simulink model "ASM_Traffic_V2X_Complete_Model_2"  (R2019a)
settings: Solver=ode1  StartTime=SIM.tstart.v  StopTime=Inf  FixedStep=SIM.StepSize.v  RelTol=1e-3
PostLoadFcn:
  | if any(exist('dsrtsu_mdlpostloadfcn', 'file') ~= 0), dsrtsu_mdlpostloadfcn('Execute', bdroot); end
  | try, asm_mdl_postloadfcn(bdroot, 'UpdateModel', 2200); catch, disp(lasterr); end,
undefined symbols (not defined in the file): _SensorPnts_1, _SensorPnts_13, _SensorPnts_17, _SensorPnts_21, _SensorPnts_25, _SensorPnts_29, _SensorPnts_33, _SensorPnts_37, _SensorPnts_41, _SensorPnts_45, _SensorPnts_49, _SensorPnts_5, _SensorPnts_53, _SensorPnts_57, _SensorPnts_9, _to_, CPT, G5A, ITS, MDL, rad, s_to_rpm, SIM
libraries: simulink x169, ASM_VehicleDynamics_lib x126, ASM_Traffic_lib x83, ASM_Utils_lib x49, mdbs x45, ASM_Environment_lib x17, dspindex x12, dsaV2xLibraryAux x10, dsmpblib x6, dsaV2xAsn1Library x4, dsaV2xLibrary x4, ASM_BrakeHydraulics_lib x4
(part 33 of 36)

== system ASM_Traffic_V2X_Complete_Model_2/MDLUserInterface/Environment/MDL_DISP/Traffic/Object_Sensor_2D/IdxSelect_2DSensor/Scopezone_Element_Data_Selection3/Object_Type[]1 ==
  In1 : Inport
  Out1 : Outport
  wires:
  In1/1 -> Out1/1

== system ASM_Traffic_V2X_Complete_Model_2/MDLUserInterface/Environment/MDL_DISP/Traffic/Object_Sensor_2D/IdxSelect_2DSensor/Scopezone_Element_Data_Selection3/a_Rel[m|s2]1 ==
  In1 : Inport
  Out1 : Outport
  wires:
  In1/1 -> Out1/1

== system ASM_Traffic_V2X_Complete_Model_2/MDLUserInterface/Environment/MDL_DISP/Traffic/Object_Sensor_2D/IdxSelect_2DSensor/Scopezone_Element_Data_Selection3/v_Rel[m|s]1 ==
  In1 : Inport
  Out1 : Outport
  wires:
  In1/1 -> Out1/1

== system ASM_Traffic_V2X_Complete_Model_2/MDLUserInterface/Environment/MDL_DISP/Traffic/Object_Sensor_2D/IdxSelect_2DSensor/Scopezone_Element_Data_Selection4/Angle_Hor_Rel[deg]1 ==
  In1 : Inport
  Out1 : Outport
  wires:
  In1/1 -> Out1/1

== system ASM_Traffic_V2X_Complete_Model_2/MDLUserInterface/Environment/MDL_DISP/Traffic/Object_Sensor_2D/IdxSelect_2DSensor/Scopezone_Element_Data_Selection4/Distance[m]1 ==
  In1 : Inport
  Out1 : Outport
  wires:
  In1/1 -> Out1/1

== system ASM_Traffic_V2X_Complete_Model_2/MDLUserInterface/Environment/MDL_DISP/Traffic/Object_Sensor_2D/IdxSelect_2DSensor/Scopezone_Element_Data_Selection4/Flag_Object_In_Scope[0Out|1In]1 ==
  In1 : Inport
  Out1 : Outport
  wires:
  In1/1 -> Out1/1

== system ASM_Traffic_V2X_Complete_Model_2/MDLUserInterface/Environment/MDL_DISP/Traffic/Object_Sensor_2D/IdxSelect_2DSensor/Scopezone_Element_Data_Selection4/Flag_Sensor_Apex_In_Object[0Out|1In]1 ==
  In1 : Inport
  Out1 : Outport
  wires:
  In1/1 -> Out1/1

== system ASM_Traffic_V2X_Complete_Model_2/MDLUserInterface/Environment/MDL_DISP/Traffic/Object_Sensor_2D/IdxSelect_2DSensor/Scopezone_Element_Data_Selection4/Height_Max[m]1 ==
  In1 : Inport
  Out1 : Outport
  wires:
  In1/1 -> Out1/1

== system ASM_Traffic_V2X_Complete_Model_2/MDLUserInterface/Environment/MDL_DISP/Traffic/Object_Sensor_2D/IdxSelect_2DSensor/Scopezone_Element_Data_Selection4/Height_Min[m]1 ==
  In1 : Inport
  Out1 : Outport
  wires:
  In1/1 -> Out1/1

== system ASM_Traffic_V2X_Complete_Model_2/MDLUserInterface/Environment/MDL_DISP/Traffic/Object_Sensor_2D/IdxSelect_2DSensor/Scopezone_Element_Data_Selection4/Object_ID[]1 ==
  In1 : Inport
  Out1 : Outport
  wires:
  In1/1 -> Out1/1

== system ASM_Traffic_V2X_Complete_Model_2/MDLUserInterface/Environment/MDL_DISP/Traffic/Object_Sensor_2D/IdxSelect_2DSensor/Scopezone_Element_Data_Selection4/Object_Type[]1 ==
  In1 : Inport
  Out1 : Outport
  wires:
  In1/1 -> Out1/1

== system ASM_Traffic_V2X_Complete_Model_2/MDLUserInterface/Environment/MDL_DISP/Traffic/Object_Sensor_2D/IdxSelect_2DSensor/Scopezone_Element_Data_Selection4/a_Rel[m|s2]1 ==
  In1 : Inport
  Out1 : Outport
  wires:
  In1/1 -> Out1/1

== system ASM_Traffic_V2X_Complete_Model_2/MDLUserInterface/Environment/MDL_DISP/Traffic/Object_Sensor_2D/IdxSelect_2DSensor/Scopezone_Element_Data_Selection4/v_Rel[m|s]1 ==
  In1 : Inport
  Out1 : Outport
  wires:
  In1/1 -> Out1/1

== system ASM_Traffic_V2X_Complete_Model_2/MDLUserInterface/Environment/MDL_DISP/Traffic/Object_Sensor_2D/IdxSelect_2DSensor/Scopezone_Element_Data_Selection5/Angle_Hor_Rel[deg]1 ==
  In1 : Inport
  Out1 : Outport
  wires:
  In1/1 -> Out1/1

== system ASM_Traffic_V2X_Complete_Model_2/MDLUserInterface/Environment/MDL_DISP/Traffic/Object_Sensor_2D/IdxSelect_2DSensor/Scopezone_Element_Data_Selection5/Distance[m]1 ==
  In1 : Inport
  Out1 : Outport
  wires:
  In1/1 -> Out1/1

== system ASM_Traffic_V2X_Complete_Model_2/MDLUserInterface/Environment/MDL_DISP/Traffic/Object_Sensor_2D/IdxSelect_2DSensor/Scopezone_Element_Data_Selection5/Flag_Object_In_Scope[0Out|1In]1 ==
  In1 : Inport
  Out1 : Outport
  wires:
  In1/1 -> Out1/1

== system ASM_Traffic_V2X_Complete_Model_2/MDLUserInterface/Environment/MDL_DISP/Traffic/Object_Sensor_2D/IdxSelect_2DSensor/Scopezone_Element_Data_Selection5/Flag_Sensor_Apex_In_Object[0Out|1In]1 ==
  In1 : Inport
  Out1 : Outport
  wires:
  In1/1 -> Out1/1

== system ASM_Traffic_V2X_Complete_Model_2/MDLUserInterface/Environment/MDL_DISP/Traffic/Object_Sensor_2D/IdxSelect_2DSensor/Scopezone_Element_Data_Selection5/Height_Max[m]1 ==
  In1 : Inport
  Out1 : Outport
  wires:
  In1/1 -> Out1/1

== system ASM_Traffic_V2X_Complete_Model_2/MDLUserInterface/Environment/MDL_DISP/Traffic/Object_Sensor_2D/IdxSelect_2DSensor/Scopezone_Element_Data_Selection5/Height_Min[m]1 ==
  In1 : Inport
  Out1 : Outport
  wires:
  In1/1 -> Out1/1

== system ASM_Traffic_V2X_Complete_Model_2/MDLUserInterface/Environment/MDL_DISP/Traffic/Object_Sensor_2D/IdxSelect_2DSensor/Scopezone_Element_Data_Selection5/Object_ID[]1 ==
  In1 : Inport
  Out1 : Outport
  wires:
  In1/1 -> Out1/1

== system ASM_Traffic_V2X_Complete_Model_2/MDLUserInterface/Environment/MDL_DISP/Traffic/Object_Sensor_2D/IdxSelect_2DSensor/Scopezone_Element_Data_Selection5/Object_Type[]1 ==
  In1 : Inport
  Out1 : Outport
  wires:
  In1/1 -> Out1/1

== system ASM_Traffic_V2X_Complete_Model_2/MDLUserInterface/Environment/MDL_DISP/Traffic/Object_Sensor_2D/IdxSelect_2DSensor/Scopezone_Element_Data_Selection5/a_Rel[m|s2]1 ==
  In1 : Inport
  Out1 : Outport
  wires:
  In1/1 -> Out1/1

== system ASM_Traffic_V2X_Complete_Model_2/MDLUserInterface/Environment/MDL_DISP/Traffic/Object_Sensor_2D/IdxSelect_2DSensor/Scopezone_Element_Data_Selection5/v_Rel[m|s]1 ==
  In1 : Inport
  Out1 : Outport
  wires:
  In1/1 -> Out1/1

== system ASM_Traffic_V2X_Complete_Model_2/MDLUserInterface/Environment/MDL_DISP/Traffic/Traffic_Sign_Sensor/GetTrfSgnDataByIndex_1/SwitchObjectPosition/Idx_comp ==
  Idx : Inport
  Add : Sum
  Add1 : Sum  Inputs=+-
  Add2 : Sum
  Add3 : Sum
  Constant : Constant
  Constant1 : Constant
  Constant2 : Constant  Value=2
  Constant3 : Constant  Value=3
  Gain : Gain  Gain=3
  Idx_comp_x : Outport
  Idx_comp_y : Outport  Port=2
  Idx_comp_z : Outport  Port=3
  wires:
  Constant/1 -> Add/2
  Idx/1 -> Add1/1
  Constant1/1 -> Add1/2
  Add1/1 -> Gain/1
  Gain/1 -> Add3/1, Add2/1, Add/1
  Add/1 -> Idx_comp_x/1
  Constant2/1 -> Add2/2
  Constant3/1 -> Add3/2
  Add2/1 -> Idx_comp_y/1
  Add3/1 -> Idx_comp_z/1

== system ASM_Traffic_V2X_Complete_Model_2/MDLUserInterface/Environment/MDL_DISP/Traffic/Traffic_Sign_Sensor/GetTrfSgnDataByIndex_1/SwitchObjectPosition/Idx_comp1 ==
  Idx : Inport
  Add : Sum
  Add1 : Sum  Inputs=+-
  Add2 : Sum
  Add3 : Sum
  Constant : Constant
  Constant1 : Constant
  Constant2 : Constant  Value=2
  Constant3 : Constant  Value=3
  Gain : Gain  Gain=3
  Idx_comp_x : Outport
  Idx_comp_y : Outport  Port=2
  Idx_comp_z : Outport  Port=3
  wires:
  Add3/1 -> Idx_comp_z/1
  Add2/1 -> Idx_comp_y/1
  Constant3/1 -> Add3/2
  Constant2/1 -> Add2/2
  Add/1 -> Idx_comp_x/1
  Gain/1 -> Add/1, Add2/1, Add3/1
  Add1/1 -> Gain/1
  Constant1/1 -> Add1/2
  Idx/1 -> Add1/1
  Constant/1 -> Add/2

== system ASM_Traffic_V2X_Complete_Model_2/MDLUserInterface/Environment/MDL_DISP/Traffic/Traffic_Sign_Sensor/GetTrfSgnDataByIndex_1/SwitchObjectPosition/Idx_comp2 ==
  Idx : Inport
  Add : Sum
  Add1 : Sum  Inputs=+-
  Add2 : Sum
  Add3 : Sum
  Constant : Constant
  Constant1 : Constant
  Constant2 : Constant  Value=2
  Constant3 : Constant  Value=3
  Gain : Gain  Gain=3
  Idx_comp_x : Outport
  Idx_comp_y : Outport  Port=2
  Idx_comp_z : Outport  Port=3
  wires:
  Constant/1 -> Add/2
  Idx/1 -> Add1/1
  Constant1/1 -> Add1/2
  Add1/1 -> Gain/1
  Gain/1 -> Add3/1, Add2/1, Add/1
  Add/1 -> Idx_comp_x/1
  Constant2/1 -> Add2/2
  Constant3/1 -> Add3/2
  Add2/1 -> Idx_comp_y/1
  Add3/1 -> Idx_comp_z/1

== system ASM_Traffic_V2X_Complete_Model_2/MDLUserInterface/Environment/MDL_DISP/Traffic/Traffic_Sign_Sensor/GetTrfSgnDataByIndex_1/SwitchSignProperties/Idx_comp ==
  Idx : Inport
  Add{,2..5} (5 alike) : Sum
  Add1 : Sum  Inputs=+-
  Constant : Constant
  Constant1 : Constant
  Constant2 : Constant  Value=2
  Constant3 : Constant  Value=3
  Constant4 : Constant  Value=4
  Constant5 : Constant  Value=5
  Gain : Gain  Gain=5
  Idx_comp_1 : Outport
  Idx_comp_2 : Outport  Port=2
  Idx_comp_3 : Outport  Port=3
  Idx_comp_4 : Outport  Port=4
  Idx_comp_5 : Outport  Port=5
  wires:
  Constant/1 -> Add/2
  Idx/1 -> Add1/1
  Constant1/1 -> Add1/2
  Add1/1 -> Gain/1
  Add/1 -> Idx_comp_1/1
  Constant2/1 -> Add2/2
  Constant3/1 -> Add3/2
  Add2/1 -> Idx_comp_2/1
  Add3/1 -> Idx_comp_3/1
  Gain/1 -> Add5/1, Add4/1, Add3/1, Add2/1, Add/1
  Constant4/1 -> Add4/2
  Constant5/1 -> Add5/2
  Add4/1 -> Idx_comp_4/1
  Add5/1 -> Idx_comp_5/1

== system ASM_Traffic_V2X_Complete_Model_2/MDLUserInterface/MotionDeskInterface/MOTION_DESK_INTERFACE/Traffic_Animation/Sensors_Animation/Sensor_Points/Object_Sensor_2D_Points/Calc_Object_Sensor_2D_Points ==
  Transform_In : Inport
  ModelSignals : Inport  Port=2
  Bus Selector2 : BusSelector  OutputSignals=Angle_Hor_Rel[deg],Distance[m],Num_SensorRays_Used[]
  Sensor_Points : Subsystem
  AnimationSignals : Outport
  wires:
  Bus Selector2/1 -> Sensor_Points/2(Angle_Hor_Rel[deg])  "<Angle_Hor_Rel[deg]>"
  Bus Selector2/3 -> Sensor_Points/4(Num_SensorRays_Used[])  "<Num_SensorRays_Used[]>"
  Sensor_Points/1(Translate[x;y;z][m]) -> AnimationSignals/1
  Bus Selector2/2 -> Sensor_Points/3(Distance[m])  "<Distance[m]>"
  Transform_In/1 -> Sensor_Points/1(Transform_In)
  ModelSignals/1 -> Bus Selector2/1

== system ASM_Traffic_V2X_Complete_Model_2/MDLUserInterface/MotionDeskInterface/MOTION_DESK_INTERFACE/Traffic_Animation/Sensors_Animation/Sensor_Points/Object_Sensor_2D_Points/Object_Sensor_2D_Transformation ==
  Transform_In1 : Inport
  ModelSignals : Inport  Port=2
  Bus Selector1 : BusSelector  OutputSignals=Pos_Sensor_Apex_CoorSys_V[x;y;z][m],Angle_z_Orientation_Sensor_CoorSys_V[deg]
  MD_Object : mdbs/MD_Object  strObjId=38  strObjName=Object_Senor_2D  strBlockType=TRANS  bGUIEventOK=0
      settings: SourceProductName=dSPACE MotionDesk Blockset
  Mux : Mux  Inputs=3
  zero : Constant  Value=0
  Transform_Out : Outport
  wires:
  Bus Selector1/2 -> Mux/1  "<Angle_z_Orientation_Sensor_CoorSys_V[deg]>"
  Transform_In1/1 -> MD_Object/1
  Mux/1 -> MD_Object/3
  zero/1 -> Mux/2, Mux/3
  Bus Selector1/1 -> MD_Object/2  "<Pos_Sensor_Apex_CoorSys_V[x;y;z][m]>"
  ModelSignals/1 -> Bus Selector1/1
  MD_Object/1 -> Transform_Out/1

== system ASM_Traffic_V2X_Complete_Model_2/MDLUserInterface/MotionDeskInterface/MOTION_DESK_INTERFACE/Traffic_Animation/Sensors_Animation/Sensor_Points/Object_Sensor_3D_CustomPoints/AdaptPointSensor1_To_Dim_60 ==
  ID[] : Inport
  Pos_ObjectPoint_CoorSys_E[x;y;z][m] : Inport  Port=2
  Demux1 : Demux  Outputs=3
  Mux1 : Mux  Inputs=3
  Select_1_60_{1..4} (4 alike) : Selector  InputPortWidth=MDL.Traffic.Sensors.CustomPoints_1.Const_Output_Dimension_Object_Points.v*MDL.Traffic.Sensors.CustomPoints_1.Const_Output_Dimension_Objects.v  IndexOptions=Index vector (dialog)  Indices=[1:60]  OutputSizes=1
  ID_Adatpted[] : Outport
  Pos_ObjectPoint_CoorSys_E_Adapted[x;y;z][m] : Outport  Port=2
  wires:
  Pos_ObjectPoint_CoorSys_E[x;y;z][m]/1 -> Demux1/1
  ID[]/1 -> Select_1_60_1/1
  Select_1_60_1/1 -> ID_Adatpted[]/1
  Select_1_60_2/1 -> Mux1/1
  Demux1/1 -> Select_1_60_2/1
  Demux1/2 -> Select_1_60_3/1
  Select_1_60_3/1 -> Mux1/2
  Select_1_60_4/1 -> Mux1/3
  Demux1/3 -> Select_1_60_4/1
  Mux1/1 -> Pos_ObjectPoint_CoorSys_E_Adapted[x;y;z][m]/1

== system ASM_Traffic_V2X_Complete_Model_2/MDLUserInterface/MotionDeskInterface/MOTION_DESK_INTERFACE/Traffic_Animation/Sensors_Animation/Sensor_Points/Object_Sensor_3D_CustomPoints/AdaptPointSensor2_To_Dim_60 ==
  ID[] : Inport
  Pos_ObjectPoint_CoorSys_E[x;y;z][m] : Inport  Port=2
  Demux1 : Demux  Outputs=3
  Mux1 : Mux  Inputs=3
  Select_1_60_{1..4} (4 alike) : Selector  InputPortWidth=MDL.Traffic.Sensors.CustomPoints_2.Const_Output_Dimension_Object_Points.v*MDL.Traffic.Sensors.CustomPoints_2.Const_Output_Dimension_Objects.v  IndexOptions=Index vector (dialog)  Indices=[1:60]  OutputSizes=1
  ID_Adatpted[] : Outport
  Pos_ObjectPoint_CoorSys_E_Adapted[x;y;z][m] : Outport  Port=2
  wires:
  Demux1/2 -> Select_1_60_3/1
  Demux1/3 -> Select_1_60_4/1
  ID[]/1 -> Select_1_60_1/1
  Pos_ObjectPoint_CoorSys_E[x;y;z][m]/1 -> Demux1/1
  Mux1/1 -> Pos_ObjectPoint_CoorSys_E_Adapted[x;y;z][m]/1
  Demux1/1 -> Select_1_60_2/1
  Select_1_60_1/1 -> ID_Adatpted[]/1
  Select_1_60_2/1 -> Mux1/1
  Select_1_60_3/1 -> Mux1/2
  Select_1_60_4/1 -> Mux1/3

== system ASM_Traffic_V2X_Complete_Model_2/MDLUserInterface/MotionDeskInterface/MOTION_DESK_INTERFACE/Traffic_Animation/Sensors_Animation/Sensor_Points/Object_Sensor_3D_CustomPoints/AdaptPointSensor3_To_Dim_60 ==
  ID[] : Inport
  Pos_ObjectPoint_CoorSys_E[x;y;z][m] : Inport  Port=2
  Demux1 : Demux  Outputs=3
  Mux1 : Mux  Inputs=3
  Select_1_60_{1..4} (4 alike) : Selector  InputPortWidth=MDL.Traffic.Sensors.CustomPoints_3.Const_Output_Dimension_Object_Points.v*MDL.Traffic.Sensors.CustomPoints_3.Const_Output_Dimension_Objects.v  IndexOptions=Index vector (dialog)  Indices=[1:60]  OutputSizes=1
  ID_Adatpted[] : Outport
  Pos_ObjectPoint_CoorSys_E_Adapted[x;y;z][m] : Outport  Port=2
  wires:
  Demux1/1 -> Select_1_60_2/1
  Mux1/1 -> Pos_ObjectPoint_CoorSys_E_Adapted[x;y;z][m]/1
  Pos_ObjectPoint_CoorSys_E[x;y;z][m]/1 -> Demux1/1
  ID[]/1 -> Select_1_60_1/1
  Demux1/3 -> Select_1_60_4/1
  Demux1/2 -> Select_1_60_3/1
  Select_1_60_1/1 -> ID_Adatpted[]/1
  Select_1_60_2/1 -> Mux1/1
  Select_1_60_3/1 -> Mux1/2
  Select_1_60_4/1 -> Mux1/3

== system ASM_Traffic_V2X_Complete_Model_2/MDLUserInterface/MotionDeskInterface/MOTION_DESK_INTERFACE/Traffic_Animation/Sensors_Animation/Sensor_Points/Object_Sensor_3D_RadarEffect_Points/AdaptPointDimensionSensor1 ==
  ID[] : Inport
  Pos_ObjectPoint_CoorSys_E[x;y;z][m] : Inport  Port=2
  Demux1 : Demux  Outputs=3
  Mux1 : Mux  Inputs=3
  Selector{1..4} (4 alike) : Selector  InputPortWidth=MDL.Traffic.Sensors.CustomPoints_1.Const_Output_Dimension_Object_Points.v*MDL.Traffic.Sensors.CustomPoints_1.Const_Output_Dimension_Objects.v  IndexOptions=Index vector (dialog)  Indices=[1:60]  OutputSizes=1
  ID_Adatpted[] : Outport
  Pos_ObjectPoint_CoorSys_E_Adapted[x;y;z][m] : Outport  Port=2
  wires:
  Mux1/1 -> Pos_ObjectPoint_CoorSys_E_Adapted[x;y;z][m]/1
  Demux1/3 -> Selector4/1
  Selector4/1 -> Mux1/3
  Selector2/1 -> Mux1/2
  Demux1/2 -> Selector2/1
  Demux1/1 -> Selector1/1
  Selector1/1 -> Mux1/1
  Selector3/1 -> ID_Adatpted[]/1
  ID[]/1 -> Selector3/1
  Pos_ObjectPoint_CoorSys_E[x;y;z][m]/1 -> Demux1/1

== system ASM_Traffic_V2X_Complete_Model_2/MDLUserInterface/MotionDeskInterface/MOTION_DESK_INTERFACE/Traffic_Animation/Sensors_Animation/Sensor_Points/Object_Sensor_3D_RadarEffect_Points/AdaptPointDimensionSensor2 ==
  ID[] : Inport
  Pos_ObjectPoint_CoorSys_E[x;y;z][m] : Inport  Port=2
  Demux1 : Demux  Outputs=3
  Mux1 : Mux  Inputs=3
  Selector{1..4} (4 alike) : Selector  InputPortWidth=MDL.Traffic.Sensors.CustomPoints_2.Const_Output_Dimension_Object_Points.v*MDL.Traffic.Sensors.CustomPoints_2.Const_Output_Dimension_Objects.v  IndexOptions=Index vector (dialog)  Indices=[1:60]  OutputSizes=1
  ID_Adatpted[] : Outport
  Pos_ObjectPoint_CoorSys_E_Adapted[x;y;z][m] : Outport  Port=2
  wires:
  Selector4/1 -> Mux1/3
  Selector2/1 -> Mux1/2
  Selector1/1 -> Mux1/1
  Selector3/1 -> ID_Adatpted[]/1
  Demux1/1 -> Selector1/1
  Mux1/1 -> Pos_ObjectPoint_CoorSys_E_Adapted[x;y;z][m]/1
  Pos_ObjectPoint_CoorSys_E[x;y;z][m]/1 -> Demux1/1
  ID[]/1 -> Selector3/1
  Demux1/3 -> Selector4/1
  Demux1/2 -> Selector2/1

== system ASM_Traffic_V2X_Complete_Model_2/MDLUserInterface/MotionDeskInterface/MOTION_DESK_INTERFACE/Traffic_Animation/Sensors_Animation/Sensor_Points/Object_Sensor_3D_RadarEffect_Points/AdaptPointDimensionSensor3 ==
  ID[] : Inport
  Pos_ObjectPoint_CoorSys_E[x;y;z][m] : Inport  Port=2
  Demux1 : Demux  Outputs=3
  Mux1 : Mux  Inputs=3
  Selector{1..4} (4 alike) : Selector  InputPortWidth=MDL.Traffic.Sensors.CustomPoints_3.Const_Output_Dimension_Object_Points.v*MDL.Traffic.Sensors.CustomPoints_3.Const_Output_Dimension_Objects.v  IndexOptions=Index vector (dialog)  Indices=[1:60]  OutputSizes=1
  ID_Adatpted[] : Outport
  Pos_ObjectPoint_CoorSys_E_Adapted[x;y;z][m] : Outport  Port=2
  wires:
  Selector4/1 -> Mux1/3
  Selector3/1 -> Mux1/2
  Selector2/1 -> Mux1/1
  Selector1/1 -> ID_Adatpted[]/1
  Demux1/2 -> Selector3/1
  Demux1/3 -> Selector4/1
  ID[]/1 -> Selector1/1
  Pos_ObjectPoint_CoorSys_E[x;y;z][m]/1 -> Demux1/1
  Mux1/1 -> Pos_ObjectPoint_CoorSys_E_Adapted[x;y;z][m]/1
  Demux1/1 -> Selector2/1

== system ASM_Traffic_V2X_Complete_Model_2/IO/I//O_Subsystem/Bus Configuration (1) - In/Simulated ECUs/DrivekitCAN/Drivekit/TX/PDUs/BRAKE_REPORT ==
  PDU Features : Subsystem
  _BRAKE_REPORT_ : BusCreator  Inputs=5
  brake_dtcs : Subsystem
  brake_operator_override : Subsystem
  brake_report_enabled : Subsystem
  brake_report_magic : Subsystem
  BRAKE_REPORT : Outport
  wires:
  _BRAKE_REPORT_/1 -> BRAKE_REPORT/1  "BRAKE_REPORT"
  PDU Features/1(PDU Features) -> _BRAKE_REPORT_/1  "PDU Features"
  brake_report_magic/1(brake_report_magic) -> _BRAKE_REPORT_/2  "brake_report_magic"
  brake_report_enabled/1(brake_report_enabled) -> _BRAKE_REPORT_/3  "brake_report_enabled"
  brake_operator_override/1(brake_operator_override) -> _BRAKE_REPORT_/4  "brake_operator_override"
  brake_dtcs/1(brake_dtcs) -> _BRAKE_REPORT_/5  "brake_dtcs"

== system ASM_Traffic_V2X_Complete_Model_2/IO/I//O_Subsystem/Bus Configuration (1) - In/Simulated ECUs/DrivekitCAN/Drivekit/TX/PDUs/CHASSIS_CONTROL_REPORT ==
  PDU Features : Subsystem
  _CHASSIS_CONTROL_REPORT_ : BusCreator  Inputs=8
  front_wipers : Subsystem
  headlamps : Subsystem
  horn : Subsystem
  left_signal : Subsystem
  rear_wiper : Subsystem
  right_signal : Subsystem
  vin_request : Subsystem
  CHASSIS_CONTROL_REPORT : Outport
  wires:
  _CHASSIS_CONTROL_REPORT_/1 -> CHASSIS_CONTROL_REPORT/1  "CHASSIS_CONTROL_REPORT"
  PDU Features/1(PDU Features) -> _CHASSIS_CONTROL_REPORT_/1  "PDU Features"
  front_wipers/1(front_wipers) -> _CHASSIS_CONTROL_REPORT_/2  "front_wipers"
  rear_wiper/1(rear_wiper) -> _CHASSIS_CONTROL_REPORT_/3  "rear_wiper"
  right_signal/1(right_signal) -> _CHASSIS_CONTROL_REPORT_/4  "right_signal"
  left_signal/1(left_signal) -> _CHASSIS_CONTROL_REPORT_/5  "left_signal"
  horn/1(horn) -> _CHASSIS_CONTROL_REPORT_/6  "horn"
  vin_request/1(vin_request) -> _CHASSIS_CONTROL_REPORT_/7  "vin_request"
  headlamps/1(headlamps) -> _CHASSIS_CONTROL_REPORT_/8  "headlamps"

== system ASM_Traffic_V2X_Complete_Model_2/IO/I//O_Subsystem/Bus Configuration (1) - In/Simulated ECUs/DrivekitCAN/Drivekit/TX/PDUs/ESP12 ==
  CYL_PRES : Subsystem
  CYL_PRESS_DIAG : Subsystem
  CYL_PRES_STAT : Subsystem
  ESP12_AliveCounter : Subsystem
  ESP12_Checksum : Subsystem
  LAT_ACCEL : Subsystem
  LAT_ACCEL_DIAG : Subsystem
  LAT_ACCEL_STAT : Subsystem
  LONG_ACCEL : Subsystem
  LONG_ACCEL_DIAG : Subsystem
  LONG_ACCEL_STAT : Subsystem
  PDU Features : Subsystem
  YAW_RATE : Subsystem
  YAW_RATE_DIAG : Subsystem
  YAW_RATE_STAT : Subsystem
  _ESP12_ : BusCreator  Inputs=15
  ESP12 : Outport
  wires:
  _ESP12_/1 -> ESP12/1  "ESP12"
  PDU Features/1(PDU Features) -> _ESP12_/1  "PDU Features"
  YAW_RATE_STAT/1(YAW_RATE_STAT) -> _ESP12_/2  "YAW_RATE_STAT"
  YAW_RATE_DIAG/1(YAW_RATE_DIAG) -> _ESP12_/3  "YAW_RATE_DIAG"
  YAW_RATE/1(YAW_RATE) -> _ESP12_/4  "YAW_RATE"
  LONG_ACCEL_STAT/1(LONG_ACCEL_STAT) -> _ESP12_/5  "LONG_ACCEL_STAT"
  LONG_ACCEL_DIAG/1(LONG_ACCEL_DIAG) -> _ESP12_/6  "LONG_ACCEL_DIAG"
  LONG_ACCEL/1(LONG_ACCEL) -> _ESP12_/7  "LONG_ACCEL"
  LAT_ACCEL_STAT/1(LAT_ACCEL_STAT) -> _ESP12_/8  "LAT_ACCEL_STAT"
  LAT_ACCEL_DIAG/1(LAT_ACCEL_DIAG) -> _ESP12_/9  "LAT_ACCEL_DIAG"
  LAT_ACCEL/1(LAT_ACCEL) -> _ESP12_/10  "LAT_ACCEL"
  ESP12_Checksum/1(ESP12_Checksum) -> _ESP12_/11  "ESP12_Checksum"
  ESP12_AliveCounter/1(ESP12_AliveCounter) -> _ESP12_/12  "ESP12_AliveCounter"
  CYL_PRESS_DIAG/1(CYL_PRESS_DIAG) -> _ESP12_/13  "CYL_PRESS_DIAG"
  CYL_PRES_STAT/1(CYL_PRES_STAT) -> _ESP12_/14  "CYL_PRES_STAT"
  CYL_PRES/1(CYL_PRES) -> _ESP12_/15  "CYL_PRES"

== system ASM_Traffic_V2X_Complete_Model_2/IO/I//O_Subsystem/Bus Configuration (1) - In/Simulated ECUs/DrivekitCAN/Drivekit/TX/PDUs/FAULT_REPORT ==
  PDU Features : Subsystem
  _FAULT_REPORT_ : BusCreator  Inputs=4
  fault_dtcs : Subsystem
  fault_origin_id : Subsystem
  fault_report_magic : Subsystem
  FAULT_REPORT : Outport
  wires:
  _FAULT_REPORT_/1 -> FAULT_REPORT/1  "FAULT_REPORT"
  PDU Features/1(PDU Features) -> _FAULT_REPORT_/1  "PDU Features"
  fault_report_magic/1(fault_report_magic) -> _FAULT_REPORT_/2  "fault_report_magic"
  fault_origin_id/1(fault_origin_id) -> _FAULT_REPORT_/3  "fault_origin_id"
  fault_dtcs/1(fault_dtcs) -> _FAULT_REPORT_/4  "fault_dtcs"

== system ASM_Traffic_V2X_Complete_Model_2/IO/I//O_Subsystem/Bus Configuration (1) - In/Simulated ECUs/DrivekitCAN/Drivekit/TX/PDUs/GPS_HEADING ==
  Input : Inport
  Heading : Subsystem
  PDU Features : Subsystem
  _GPS_HEADING_ : BusCreator  Inputs=2
  GPS_HEADING : Outport
  wires:
  _GPS_HEADING_/1 -> GPS_HEADING/1  "GPS_HEADING"
  PDU Features/1(PDU Features) -> _GPS_HEADING_/1  "PDU Features"
  Heading/1(Heading) -> _GPS_HEADING_/2  "Heading"
  Input/1 -> Heading/1(Input)

== system ASM_Traffic_V2X_Complete_Model_2/IO/I//O_Subsystem/Bus Configuration (1) - In/Simulated ECUs/DrivekitCAN/Drivekit/TX/PDUs/GPS_LAT ==
  Input : Inport
  Lat : Subsystem
  PDU Features : Subsystem
  _GPS_LAT_ : BusCreator  Inputs=2
  GPS_LAT : Outport
  wires:
  _GPS_LAT_/1 -> GPS_LAT/1  "GPS_LAT"
  PDU Features/1(PDU Features) -> _GPS_LAT_/1  "PDU Features"
  Lat/1(Lat) -> _GPS_LAT_/2  "Lat"
  Input/1 -> Lat/1(Input)

== system ASM_Traffic_V2X_Complete_Model_2/IO/I//O_Subsystem/Bus Configuration (1) - In/Simulated ECUs/DrivekitCAN/Drivekit/TX/PDUs/GPS_LONG ==
  Input : Inport
  Long : Subsystem
  PDU Features : Subsystem
  _GPS_LONG_ : BusCreator  Inputs=2
  GPS_LONG : Outport
  wires:
  _GPS_LONG_/1 -> GPS_LONG/1  "GPS_LONG"
  PDU Features/1(PDU Features) -> _GPS_LONG_/1  "PDU Features"
  Long/1(Long) -> _GPS_LONG_/2  "Long"
  Input/1 -> Long/1(Input)

== system ASM_Traffic_V2X_Complete_Model_2/IO/I//O_Subsystem/Bus Configuration (1) - In/Simulated ECUs/DrivekitCAN/Drivekit/TX/PDUs/LANE_REPORT ==
  Input : Inport
  Abs : Abs
  Bus Selector : BusSelector  OutputSignals=Common.LaneID_PrefLane[],LeftSide.Distance_Marker_Left[m],RightSide.Distance_Marker_Right[m]
  PDU Features : Subsystem
  _LANE_REPORT_ : BusCreator  Inputs=4
  lane_number : Subsystem
  left_marker_distance : Subsystem
  right_marker_distance : Subsystem
  LANE_REPORT : Outport
  wires:
  Input/1 -> Bus Selector/1
  PDU Features/1(PDU Features) -> _LANE_REPORT_/1  "PDU Features"
  lane_number/1(lane_number) -> _LANE_REPORT_/2  "lane_number"
  _LANE_REPORT_/1 -> LANE_REPORT/1  "LANE_REPORT"
  left_marker_distance/1(left_marker_distance) -> _LANE_REPORT_/3  "left_marker_distance"
  right_marker_distance/1(right_marker_distance) -> _LANE_REPORT_/4  "right_marker_distance"
  Bus Selector/1 -> Abs/1  "<LaneID_PrefLane[]>"
  Bus Selector/2 -> left_marker_distance/1(Input)  "<Distance_Marker_Left[m]>"
  Bus Selector/3 -> right_marker_distance/1(Input)  "<Distance_Marker_Right[m]>"
  Abs/1 -> lane_number/1(Input)

== system ASM_Traffic_V2X_Complete_Model_2/IO/I//O_Subsystem/Bus Configuration (1) - In/Simulated ECUs/DrivekitCAN/Drivekit/TX/PDUs/SAS11 ==
  Input : Inport
  Bus Selector : BusSelector  OutputSignals=SAS_Angle Value
  PDU Features : Subsystem
  SAS_Angle : Subsystem
  SAS_CheckSum : Subsystem
  SAS_MsgCount : Subsystem
  SAS_Speed : Subsystem
  SAS_Stat : Subsystem
  _SAS11_ : BusCreator  Inputs=6
  SAS11 : Outport
  wires:
  _SAS11_/1 -> SAS11/1  "SAS11"
  PDU Features/1(PDU Features) -> _SAS11_/1  "PDU Features"
  SAS_Stat/1(SAS_Stat) -> _SAS11_/2  "SAS_Stat"
  SAS_Speed/1(SAS_Speed) -> _SAS11_/3  "SAS_Speed"
  SAS_MsgCount/1(SAS_MsgCount) -> _SAS11_/4  "SAS_MsgCount"
  SAS_CheckSum/1(SAS_CheckSum) -> _SAS11_/5  "SAS_CheckSum"
  SAS_Angle/1(SAS_Angle) -> _SAS11_/6  "SAS_Angle"
  Input/1 -> Bus Selector/1
  Bus Selector/1 -> SAS_Angle/1(Input)  "<SAS_Angle Value>"

== system ASM_Traffic_V2X_Complete_Model_2/IO/I//O_Subsystem/Bus Configuration (1) - In/Simulated ECUs/DrivekitCAN/Drivekit/TX/PDUs/STEERING_ANGLE_REPORT ==
  PDU Features : Subsystem
  _STEERING_ANGLE_REPORT_ : BusCreator  Inputs=3
  steering_angle_report_errors : Subsystem
  steering_angle_report_flags : Subsystem
  STEERING_ANGLE_REPORT : Outport
  wires:
  _STEERING_ANGLE_REPORT_/1 -> STEERING_ANGLE_REPORT/1  "STEERING_ANGLE_REPORT"
  PDU Features/1(PDU Features) -> _STEERING_ANGLE_REPORT_/1  "PDU Features"
  steering_angle_report_flags/1(steering_angle_report_flags) -> _STEERING_ANGLE_REPORT_/2  "steering_angle_report_flags"
  steering_angle_report_errors/1(steering_angle_report_errors) -> _STEERING_ANGLE_REPORT_/3  "steering_angle_report_errors"

== system ASM_Traffic_V2X_Complete_Model_2/IO/I//O_Subsystem/Bus Configuration (1) - In/Simulated ECUs/DrivekitCAN/Drivekit/TX/PDUs/STEERING_REPORT ==
  PDU Features : Subsystem
  _STEERING_REPORT_ : BusCreator  Inputs=5
  steering_dtcs : Subsystem
  steering_operator_override : Subsystem
  steering_report_enabled : Subsystem
  steering_report_magic : Subsystem
  STEERING_REPORT : Outport
  wires:
  _STEERING_REPORT_/1 -> STEERING_REPORT/1  "STEERING_REPORT"
  PDU Features/1(PDU Features) -> _STEERING_REPORT_/1  "PDU Features"
  steering_report_magic/1(steering_report_magic) -> _STEERING_REPORT_/2  "steering_report_magic"
  steering_report_enabled/1(steering_report_enabled) -> _STEERING_REPORT_/3  "steering_report_enabled"
  steering_operator_override/1(steering_operator_override) -> _STEERING_REPORT_/4  "steering_operator_override"
  steering_dtcs/1(steering_dtcs) -> _STEERING_REPORT_/5  "steering_dtcs"

== system ASM_Traffic_V2X_Complete_Model_2/IO/I//O_Subsystem/Bus Configuration (1) - In/Simulated ECUs/DrivekitCAN/Drivekit/TX/PDUs/THROTTLE_REPORT ==
  PDU Features : Subsystem
  _THROTTLE_REPORT_ : BusCreator  Inputs=5
  throttle_dtcs : Subsystem
  throttle_operator_override : Subsystem
  throttle_report_enabled : Subsystem
  throttle_report_magic : Subsystem
  THROTTLE_REPORT : Outport
  wires:
  _THROTTLE_REPORT_/1 -> THROTTLE_REPORT/1  "THROTTLE_REPORT"
  PDU Features/1(PDU Features) -> _THROTTLE_REPORT_/1  "PDU Features"
  throttle_report_magic/1(throttle_report_magic) -> _THROTTLE_REPORT_/2  "throttle_report_magic"
  throttle_report_enabled/1(throttle_report_enabled) -> _THROTTLE_REPORT_/3  "throttle_report_enabled"
  throttle_operator_override/1(throttle_operator_override) -> _THROTTLE_REPORT_/4  "throttle_operator_override"
  throttle_dtcs/1(throttle_dtcs) -> _THROTTLE_REPORT_/5  "throttle_dtcs"

== system ASM_Traffic_V2X_Complete_Model_2/IO/I//O_Subsystem/Bus Configuration (1) - In/Simulated ECUs/DrivekitCAN/Drivekit/TX/PDUs/WHL_SPD11 ==
  Input : Inport
  Bus Selector : BusSelector  OutputSignals=signal2.WHL_SPD_RR Value,signal2.WHL_SPD_RL Value,signal2.WHL_SPD_FR Value,signal2.WHL_SPD_FL Value
  PDU Features : Subsystem
  WHL_SPD_AliveCounter_LSB : Subsystem
  WHL_SPD_AliveCounter_MSB : Subsystem
  WHL_SPD_Checksum_LSB : Subsystem
  WHL_SPD_Checksum_MSB : Subsystem
  WHL_SPD_FL : Subsystem
  WHL_SPD_FR : Subsystem
  WHL_SPD_RL : Subsystem
  WHL_SPD_RR : Subsystem
  _WHL_SPD11_ : BusCreator  Inputs=9
  WHL_SPD11 : Outport
  wires:
  _WHL_SPD11_/1 -> WHL_SPD11/1  "WHL_SPD11"
  PDU Features/1(PDU Features) -> _WHL_SPD11_/1  "PDU Features"
  WHL_SPD_RR/1(WHL_SPD_RR) -> _WHL_SPD11_/2  "WHL_SPD_RR"
  WHL_SPD_RL/1(WHL_SPD_RL) -> _WHL_SPD11_/3  "WHL_SPD_RL"
  WHL_SPD_FR/1(WHL_SPD_FR) -> _WHL_SPD11_/4  "WHL_SPD_FR"
  WHL_SPD_FL/1(WHL_SPD_FL) -> _WHL_SPD11_/5  "WHL_SPD_FL"
  WHL_SPD_Checksum_MSB/1(WHL_SPD_Checksum_MSB) -> _WHL_SPD11_/6  "WHL_SPD_Checksum_MSB"
  WHL_SPD_Checksum_LSB/1(WHL_SPD_Checksum_LSB) -> _WHL_SPD11_/7  "WHL_SPD_Checksum_LSB"
  WHL_SPD_AliveCounter_MSB/1(WHL_SPD_AliveCounter_MSB) -> _WHL_SPD11_/8  "WHL_SPD_AliveCounter_MSB"
  WHL_SPD_AliveCounter_LSB/1(WHL_SPD_AliveCounter_LSB) -> _WHL_SPD11_/9  "WHL_SPD_AliveCounter_LSB"
  Input/1 -> Bus Selector/1
  Bus Selector/1 -> WHL_SPD_RR/1(Input)  "<WHL_SPD_RR Value>"
  Bus Selector/2 -> WHL_SPD_RL/1(Input)  "<WHL_SPD_RL Value>"
  Bus Selector/3 -> WHL_SPD_FR/1(Input)  "<WHL_SPD_FR Value>"
  Bus Selector/4 -> WHL_SPD_FL/1(Input)  "<WHL_SPD_FL Value>"

== system ASM_Traffic_V2X_Complete_Model_2/IO/I//O_Subsystem/Bus Configuration (1) - Out/Simulated ECUs/DrivekitCAN/Drivekit/RX/PDUs/BRAKE_COMMAND ==
  BRAKE_COMMAND : Inport
  _BRAKE_COMMAND_ : BusSelector  OutputSignals=brake_command_magic,brake_pedal_command
  brake_command_magic : Subsystem
  brake_pedal_command : Subsystem
  wires:
  BRAKE_COMMAND/1 -> _BRAKE_COMMAND_/1  "BRAKE_COMMAND"
  _BRAKE_COMMAND_/1 -> brake_command_magic/1(brake_command_magic)  "<brake_command_magic>"
  _BRAKE_COMMAND_/2 -> brake_pedal_command/1(brake_pedal_command)  "<brake_pedal_command>"

== system ASM_Traffic_V2X_Complete_Model_2/IO/I//O_Subsystem/Bus Configuration (1) - Out/Simulated ECUs/DrivekitCAN/Drivekit/RX/PDUs/BRAKE_DISABLE ==
  BRAKE_DISABLE : Inport
  _BRAKE_DISABLE_ : BusSelector  OutputSignals=brake_disable_magic
  brake_disable_magic : Subsystem
  wires:
  BRAKE_DISABLE/1 -> _BRAKE_DISABLE_/1  "BRAKE_DISABLE"
  _BRAKE_DISABLE_/1 -> brake_disable_magic/1(brake_disable_magic)  "<brake_disable_magic>"

== system ASM_Traffic_V2X_Complete_Model_2/IO/I//O_Subsystem/Bus Configuration (1) - Out/Simulated ECUs/DrivekitCAN/Drivekit/RX/PDUs/BRAKE_ENABLE ==
  BRAKE_ENABLE : Inport
  _BRAKE_ENABLE_ : BusSelector  OutputSignals=brake_enable_magic
  brake_enable_magic : Subsystem
  wires:
  BRAKE_ENABLE/1 -> _BRAKE_ENABLE_/1  "BRAKE_ENABLE"
  _BRAKE_ENABLE_/1 -> brake_enable_magic/1(brake_enable_magic)  "<brake_enable_magic>"

== system ASM_Traffic_V2X_Complete_Model_2/IO/I//O_Subsystem/Bus Configuration (1) - Out/Simulated ECUs/DrivekitCAN/Drivekit/RX/PDUs/CHASSIS_CONTROL_COMMAND ==
  CHASSIS_CONTROL_COMMAND : Inport
  _CHASSIS_CONTROL_COMMAND_ : BusSelector  OutputSignals=front_wipers,rear_wiper,right_signal,left_signal,horn,vin,headlamps
  front_wipers : Subsystem
  headlamps : Subsystem
  horn : Subsystem
  left_signal : Subsystem
  rear_wiper : Subsystem
  right_signal : Subsystem
  vin : Subsystem
  wires:
  CHASSIS_CONTROL_COMMAND/1 -> _CHASSIS_CONTROL_COMMAND_/1  "CHASSIS_CONTROL_COMMAND"
  _CHASSIS_CONTROL_COMMAND_/1 -> front_wipers/1(front_wipers)  "<front_wipers>"
  _CHASSIS_CONTROL_COMMAND_/2 -> rear_wiper/1(rear_wiper)  "<rear_wiper>"
  _CHASSIS_CONTROL_COMMAND_/3 -> right_signal/1(right_signal)  "<right_signal>"
  _CHASSIS_CONTROL_COMMAND_/4 -> left_signal/1(left_signal)  "<left_signal>"
  _CHASSIS_CONTROL_COMMAND_/5 -> horn/1(horn)  "<horn>"
  _CHASSIS_CONTROL_COMMAND_/6 -> vin/1(vin)  "<vin>"
  _CHASSIS_CONTROL_COMMAND_/7 -> headlamps/1(headlamps)  "<headlamps>"

== system ASM_Traffic_V2X_Complete_Model_2/IO/I//O_Subsystem/Bus Configuration (1) - Out/Simulated ECUs/DrivekitCAN/Drivekit/RX/PDUs/STEERING_ANGLE_COMMAND ==
  STEERING_ANGLE_COMMAND : Inport
  _STEERING_ANGLE_COMMAND_ : BusSelector  OutputSignals=steering_angle_cmd_flags,steering_angle_cmd_angle,steering_angle_cmd_max_velocity
  steering_angle_cmd_angle : Subsystem
  steering_angle_cmd_flags : Subsystem
  steering_angle_cmd_max_velocity : Subsystem
  wires:
  STEERING_ANGLE_COMMAND/1 -> _STEERING_ANGLE_COMMAND_/1  "STEERING_ANGLE_COMMAND"
  _STEERING_ANGLE_COMMAND_/1 -> steering_angle_cmd_flags/1(steering_angle_cmd_flags)  "<steering_angle_cmd_flags>"
  _STEERING_ANGLE_COMMAND_/2 -> steering_angle_cmd_angle/1(steering_angle_cmd_angle)  "<steering_angle_cmd_angle>"
  _STEERING_ANGLE_COMMAND_/3 -> steering_angle_cmd_max_velocity/1(steering_angle_cmd_max_velocity)  "<steering_angle_cmd_max_velocity>"

== system ASM_Traffic_V2X_Complete_Model_2/IO/I//O_Subsystem/Bus Configuration (1) - Out/Simulated ECUs/DrivekitCAN/Drivekit/RX/PDUs/STEERING_DISABLE ==
  STEERING_DISABLE : Inport
  _STEERING_DISABLE_ : BusSelector  OutputSignals=steering_disable_magic
  steering_disable_magic : Subsystem
  wires:
  STEERING_DISABLE/1 -> _STEERING_DISABLE_/1  "STEERING_DISABLE"
  _STEERING_DISABLE_/1 -> steering_disable_magic/1(steering_disable_magic)  "<steering_disable_magic>"

== system ASM_Traffic_V2X_Complete_Model_2/IO/I//O_Subsystem/Bus Configuration (1) - Out/Simulated ECUs/DrivekitCAN/Drivekit/RX/PDUs/STEERING_ENABLE ==
  STEERING_ENABLE : Inport
  _STEERING_ENABLE_ : BusSelector  OutputSignals=steering_enable_magic
  steering_enable_magic : Subsystem
  wires:
  STEERING_ENABLE/1 -> _STEERING_ENABLE_/1  "STEERING_ENABLE"
  _STEERING_ENABLE_/1 -> steering_enable_magic/1(steering_enable_magic)  "<steering_enable_magic>"

== system ASM_Traffic_V2X_Complete_Model_2/IO/I//O_Subsystem/Bus Configuration (1) - Out/Simulated ECUs/DrivekitCAN/Drivekit/RX/PDUs/STEERING_TORQUE_COMMAND ==
  STEERING_TORQUE_COMMAND : Inport
  _STEERING_TORQUE_COMMAND_ : BusSelector  OutputSignals=steering_command_magic,steering_torque_command
  steering_command_magic : Subsystem
  steering_torque_command : Subsystem
  wires:
  STEERING_TORQUE_COMMAND/1 -> _STEERING_TORQUE_COMMAND_/1  "STEERING_TORQUE_COMMAND"
  _STEERING_TORQUE_COMMAND_/1 -> steering_command_magic/1(steering_command_magic)  "<steering_command_magic>"
  _STEERING_TORQUE_COMMAND_/2 -> steering_torque_command/1(steering_torque_command)  "<steering_torque_command>"

== system ASM_Traffic_V2X_Complete_Model_2/IO/I//O_Subsystem/Bus Configuration (1) - Out/Simulated ECUs/DrivekitCAN/Drivekit/RX/PDUs/THROTTLE_COMMAND ==
  THROTTLE_COMMAND : Inport
  _THROTTLE_COMMAND_ : BusSelector  OutputSignals=throttle_command_magic,throttle_pedal_command
  throttle_command_magic : Subsystem
  throttle_pedal_command : Subsystem
  wires:
  THROTTLE_COMMAND/1 -> _THROTTLE_COMMAND_/1  "THROTTLE_COMMAND"
  _THROTTLE_COMMAND_/1 -> throttle_command_magic/1(throttle_command_magic)  "<throttle_command_magic>"
  _THROTTLE_COMMAND_/2 -> throttle_pedal_command/1(throttle_pedal_command)  "<throttle_pedal_command>"

== system ASM_Traffic_V2X_Complete_Model_2/IO/I//O_Subsystem/Bus Configuration (1) - Out/Simulated ECUs/DrivekitCAN/Drivekit/RX/PDUs/THROTTLE_DISABLE ==
  THROTTLE_DISABLE : Inport
  _THROTTLE_DISABLE_ : BusSelector  OutputSignals=throttle_disable_magic
  throttle_disable_magic : Subsystem
  wires:
  THROTTLE_DISABLE/1 -> _THROTTLE_DISABLE_/1  "THROTTLE_DISABLE"
  _THROTTLE_DISABLE_/1 -> throttle_disable_magic/1(throttle_disable_magic)  "<throttle_disable_magic>"

== system ASM_Traffic_V2X_Complete_Model_2/IO/I//O_Subsystem/Bus Configuration (1) - Out/Simulated ECUs/DrivekitCAN/Drivekit/RX/PDUs/THROTTLE_ENABLE ==
  THROTTLE_ENABLE : Inport
  _THROTTLE_ENABLE_ : BusSelector  OutputSignals=throttle_enable_magic
  throttle_enable_magic : Subsystem
  wires:
  THROTTLE_ENABLE/1 -> _THROTTLE_ENABLE_/1  "THROTTLE_ENABLE"
  _THROTTLE_ENABLE_/1 -> throttle_enable_magic/1(throttle_enable_magic)  "<throttle_enable_magic>"

== system ASM_Traffic_V2X_Complete_Model_2/MDL/Environment/Traffic/Sensors/Object_Sensor_3D/CustomPoints/Sensor1/CustomPointsOutput/HoldSignals ==
  ResetPulse[0|1] : Inport
  CustomPoints_Signals_In[] : Inport  Port=2
  Enable : EnablePort
  Bus Selector1 : BusSelector  OutputSignals=Flag_In_Scope[0|1],Flag_Is_Occluded[0|1],ID[],Dist_CoorSys_S[m],v_CoorSys_S[m|s],a_CoorSys_S[m|s2],Pos_CoorSys_S[x;y;z][m],Pos_CoorSys_E[x;y;z][m],Angle_Hor_CoorSys_S[deg],Angle_Ver_CoorSys_S[deg],Data_1[],Data_2[],Data_3[],Data_4[],Data_5[],Object_ID[],Object_Type[]
  CUSTOM_POINTS_SIGNALS_RESET_1 : ASM_Traffic_lib/Sensors/Custom Points/CUSTOM_POINTS_SIGNALS_RESET  ASMProperties=struct('Name','CUSTOM_POINTS_SIGNALS_RESET','Version','1.0','Library','ASM_Traffic_lib')  ASMInstanceName=custom_points_signals_reset  ASMInstanceID=1
  CustomPoints_Signals_Out[] : Outport
  wires:
  CUSTOM_POINTS_SIGNALS_RESET_1/1 -> CustomPoints_Signals_Out[]/1
  ResetPulse[0|1]/1 -> CUSTOM_POINTS_SIGNALS_RESET_1/1
  Bus Selector1/5 -> CUSTOM_POINTS_SIGNALS_RESET_1/6  "<v_CoorSys_S[m|s]>"
  Bus Selector1/9 -> CUSTOM_POINTS_SIGNALS_RESET_1/10  "<Angle_Hor_CoorSys_S[deg]>"
  Bus Selector1/12 -> CUSTOM_POINTS_SIGNALS_RESET_1/13  "<Data_2[]>"
  Bus Selector1/2 -> CUSTOM_POINTS_SIGNALS_RESET_1/3  "<Flag_Is_Occluded[0|1]>"
  Bus Selector1/11 -> CUSTOM_POINTS_SIGNALS_RESET_1/12  "<Data_1[]>"
  Bus Selector1/3 -> CUSTOM_POINTS_SIGNALS_RESET_1/4  "<ID[]>"
  Bus Selector1/15 -> CUSTOM_POINTS_SIGNALS_RESET_1/16  "<Data_5[]>"
  Bus Selector1/10 -> CUSTOM_POINTS_SIGNALS_RESET_1/11  "<Angle_Ver_CoorSys_S[deg]>"
  Bus Selector1/14 -> CUSTOM_POINTS_SIGNALS_RESET_1/15  "<Data_4[]>"
  Bus Selector1/16 -> CUSTOM_POINTS_SIGNALS_RESET_1/17  "<Object_ID[]>"
  Bus Selector1/8 -> CUSTOM_POINTS_SIGNALS_RESET_1/9  "<Pos_CoorSys_E[x;y;z][m]>"
  Bus Selector1/1 -> CUSTOM_POINTS_SIGNALS_RESET_1/2  "<Flag_In_Scope[0|1]>"
  CustomPoints_Signals_In[]/1 -> Bus Selector1/1
  Bus Selector1/6 -> CUSTOM_POINTS_SIGNALS_RESET_1/7  "<a_CoorSys_S[m|s2]>"
  Bus Selector1/17 -> CUSTOM_POINTS_SIGNALS_RESET_1/18  "<Object_Type[]>"
  Bus Selector1/13 -> CUSTOM_POINTS_SIGNALS_RESET_1/14  "<Data_3[]>"
  Bus Selector1/4 -> CUSTOM_POINTS_SIGNALS_RESET_1/5  "<Dist_CoorSys_S[m]>"
  Bus Selector1/7 -> CUSTOM_POINTS_SIGNALS_RESET_1/8  "<Pos_CoorSys_S[x;y;z][m]>"

== system ASM_Traffic_V2X_Complete_Model_2/MDL/Environment/Traffic/Sensors/Object_Sensor_3D/CustomPoints/Sensor1/CustomPointsOutput/ResetPulse ==
  Enable[0|1] : Inport
  SensorActive[0|1] : Inport  Port=2
  Compare To Constant : simulink/Logic and Bit Operations/Compare To Constant  relop===  const=1  OutDataTypeStr=boolean
  Compare To Constant1 : simulink/Logic and Bit Operations/Compare To Constant  relop===  const=0  OutDataTypeStr=boolean
  Logical Operator1 : Logic  AllPortsSameDT=off  OutDataTypeStr=boolean
  Logical Operator2 : Logic  Operator=NAND  AllPortsSameDT=off  OutDataTypeStr=boolean
  Memory1 : Memory
  ResetPulse[0|1] : Outport
  wires:
  Enable[0|1]/1 -> Logical Operator2/2
  Compare To Constant1/1 -> Logical Operator1/2
  Compare To Constant/1 -> Logical Operator1/1
  Logical Operator1/1 -> ResetPulse[0|1]/1
  SensorActive[0|1]/1 -> Logical Operator2/1
  Logical Operator2/1 -> Memory1/1, Compare To Constant/1
  Memory1/1 -> Compare To Constant1/1

== system ASM_Traffic_V2X_Complete_Model_2/MDL/Environment/Traffic/Sensors/Object_Sensor_3D/CustomPoints/Sensor1/CustomPointsOutput/SignalBus ==
  CustomPoints_Signals_In[] : Inport
  Bus Creator : BusCreator  Inputs=5
  Bus Selector1 : BusSelector  OutputSignals=ID[],Object_ID[],Dist_CoorSys_S[m],Angle_Hor_CoorSys_S[deg],Pos_CoorSys_E[x;y;z][m]
  CustomPoints_Signals_Out[] : Outport
  wires:
  CustomPoints_Signals_In[]/1 -> Bus Selector1/1
  Bus Creator/1 -> CustomPoints_Signals_Out[]/1
  Bus Selector1/4 -> Bus Creator/4  "<Angle_Hor_CoorSys_S[deg]>"
  Bus Selector1/5 -> Bus Creator/5  "<Pos_CoorSys_E[x;y;z][m]>"
  Bus Selector1/2 -> Bus Creator/2  "<Object_ID[]>"
  Bus Selector1/3 -> Bus Creator/3  "<Dist_CoorSys_S[m]>"
  Bus Selector1/1 -> Bus Creator/1  "<ID[]>"

== system ASM_Traffic_V2X_Complete_Model_2/MDL/Environment/Traffic/Sensors/Object_Sensor_3D/CustomPoints/Sensor2/CustomPointsOutput/HoldSignals ==
  ResetPulse[0|1] : Inport
  CustomPoints_Signals_In[] : Inport  Port=2
  Enable : EnablePort
  Bus Selector1 : BusSelector  OutputSignals=Flag_In_Scope[0|1],Flag_Is_Occluded[0|1],ID[],Dist_CoorSys_S[m],v_CoorSys_S[m|s],a_CoorSys_S[m|s2],Pos_CoorSys_S[x;y;z][m],Pos_CoorSys_E[x;y;z][m],Angle_Hor_CoorSys_S[deg],Angle_Ver_CoorSys_S[deg],Data_1[],Data_2[],Data_3[],Data_4[],Data_5[],Object_ID[],Object_Type[]
  CUSTOM_POINTS_SIGNALS_RESET_2 : ASM_Traffic_lib/Sensors/Custom Points/CUSTOM_POINTS_SIGNALS_RESET  ASMProperties=struct('Name','CUSTOM_POINTS_SIGNALS_RESET','Version','1.0','Library','ASM_Traffic_lib')  ASMInstanceName=custom_points_signals_reset  ASMInstanceID=1
  CustomPoints_Signals_Out[] : Outport
  wires:
  Bus Selector1/12 -> CUSTOM_POINTS_SIGNALS_RESET_2/13  "<Data_2[]>"
  Bus Selector1/3 -> CUSTOM_POINTS_SIGNALS_RESET_2/4  "<ID[]>"
  Bus Selector1/17 -> CUSTOM_POINTS_SIGNALS_RESET_2/18  "<Object_Type[]>"
  Bus Selector1/16 -> CUSTOM_POINTS_SIGNALS_RESET_2/17  "<Object_ID[]>"
  Bus Selector1/5 -> CUSTOM_POINTS_SIGNALS_RESET_2/6  "<v_CoorSys_S[m|s]>"
  Bus Selector1/7 -> CUSTOM_POINTS_SIGNALS_RESET_2/8  "<Pos_CoorSys_S[x;y;z][m]>"
  Bus Selector1/8 -> CUSTOM_POINTS_SIGNALS_RESET_2/9  "<Pos_CoorSys_E[x;y;z][m]>"
  Bus Selector1/13 -> CUSTOM_POINTS_SIGNALS_RESET_2/14  "<Data_3[]>"
  ResetPulse[0|1]/1 -> CUSTOM_POINTS_SIGNALS_RESET_2/1
  Bus Selector1/4 -> CUSTOM_POINTS_SIGNALS_RESET_2/5  "<Dist_CoorSys_S[m]>"
  CUSTOM_POINTS_SIGNALS_RESET_2/1 -> CustomPoints_Signals_Out[]/1
  Bus Selector1/6 -> CUSTOM_POINTS_SIGNALS_RESET_2/7  "<a_CoorSys_S[m|s2]>"
  Bus Selector1/1 -> CUSTOM_POINTS_SIGNALS_RESET_2/2  "<Flag_In_Scope[0|1]>"
  Bus Selector1/9 -> CUSTOM_POINTS_SIGNALS_RESET_2/10  "<Angle_Hor_CoorSys_S[deg]>"
  Bus Selector1/15 -> CUSTOM_POINTS_SIGNALS_RESET_2/16  "<Data_5[]>"
  Bus Selector1/11 -> CUSTOM_POINTS_SIGNALS_RESET_2/12  "<Data_1[]>"
  Bus Selector1/14 -> CUSTOM_POINTS_SIGNALS_RESET_2/15  "<Data_4[]>"
  CustomPoints_Signals_In[]/1 -> Bus Selector1/1
  Bus Selector1/2 -> CUSTOM_POINTS_SIGNALS_RESET_2/3  "<Flag_Is_Occluded[0|1]>"
  Bus Selector1/10 -> CUSTOM_POINTS_SIGNALS_RESET_2/11  "<Angle_Ver_CoorSys_S[deg]>"

== system ASM_Traffic_V2X_Complete_Model_2/MDL/Environment/Traffic/Sensors/Object_Sensor_3D/CustomPoints/Sensor2/CustomPointsOutput/ResetPulse ==
  Enable[0|1] : Inport
  SensorActive[0|1] : Inport  Port=2
  Compare To Constant : simulink/Logic and Bit Operations/Compare To Constant  relop===  const=1  OutDataTypeStr=boolean
  Compare To Constant1 : simulink/Logic and Bit Operations/Compare To Constant  relop===  const=0  OutDataTypeStr=boolean
  Logical Operator1 : Logic  AllPortsSameDT=off  OutDataTypeStr=boolean
  Logical Operator2 : Logic  Operator=NAND  AllPortsSameDT=off  OutDataTypeStr=boolean
  Memory1 : Memory
  ResetPulse[0|1] : Outport
  wires:
  Enable[0|1]/1 -> Logical Operator2/2
  Compare To Constant1/1 -> Logical Operator1/2
  Compare To Constant/1 -> Logical Operator1/1
  Logical Operator1/1 -> ResetPulse[0|1]/1
  SensorActive[0|1]/1 -> Logical Operator2/1
  Logical Operator2/1 -> Memory1/1, Compare To Constant/1
  Memory1/1 -> Compare To Constant1/1

== system ASM_Traffic_V2X_Complete_Model_2/MDL/Environment/Traffic/Sensors/Object_Sensor_3D/CustomPoints/Sensor2/CustomPointsOutput/SignalBus ==
  CustomPoints_Signals_In[] : Inport
  Bus Creator : BusCreator  Inputs=5
  Bus Selector1 : BusSelector  OutputSignals=ID[],Object_ID[],Dist_CoorSys_S[m],Angle_Hor_CoorSys_S[deg],Pos_CoorSys_E[x;y;z][m]
  CustomPoints_Signals_Out[] : Outport
  wires:
  CustomPoints_Signals_In[]/1 -> Bus Selector1/1
  Bus Creator/1 -> CustomPoints_Signals_Out[]/1
  Bus Selector1/4 -> Bus Creator/4  "<Angle_Hor_CoorSys_S[deg]>"
  Bus Selector1/5 -> Bus Creator/5  "<Pos_CoorSys_E[x;y;z][m]>"
  Bus Selector1/2 -> Bus Creator/2  "<Object_ID[]>"
  Bus Selector1/3 -> Bus Creator/3  "<Dist_CoorSys_S[m]>"
  Bus Selector1/1 -> Bus Creator/1  "<ID[]>"

== system ASM_Traffic_V2X_Complete_Model_2/MDL/Environment/Traffic/Sensors/Object_Sensor_3D/CustomPoints/Sensor3/CustomPointsOutput/HoldSignals ==
  ResetPulse[0|1] : Inport
  CustomPoints_Signals_In[] : Inport  Port=2
  Enable : EnablePort
  Bus Selector1 : BusSelector  OutputSignals=Flag_In_Scope[0|1],Flag_Is_Occluded[0|1],ID[],Dist_CoorSys_S[m],v_CoorSys_S[m|s],a_CoorSys_S[m|s2],Pos_CoorSys_S[x;y;z][m],Pos_CoorSys_E[x;y;z][m],Angle_Hor_CoorSys_S[deg],Angle_Ver_CoorSys_S[deg],Data_1[],Data_2[],Data_3[],Data_4[],Data_5[],Object_ID[],Object_Type[]
  CUSTOM_POINTS_SIGNALS_RESET_3 : ASM_Traffic_lib/Sensors/Custom Points/CUSTOM_POINTS_SIGNALS_RESET  ASMProperties=struct('Name','CUSTOM_POINTS_SIGNALS_RESET','Version','1.0','Library','ASM_Traffic_lib')  ASMInstanceName=custom_points_signals_reset  ASMInstanceID=1
  CustomPoints_Signals_Out[] : Outport
  wires:
  Bus Selector1/3 -> CUSTOM_POINTS_SIGNALS_RESET_3/4  "<ID[]>"
  Bus Selector1/17 -> CUSTOM_POINTS_SIGNALS_RESET_3/18  "<Object_Type[]>"
  CUSTOM_POINTS_SIGNALS_RESET_3/1 -> CustomPoints_Signals_Out[]/1
  Bus Selector1/16 -> CUSTOM_POINTS_SIGNALS_RESET_3/17  "<Object_ID[]>"
  Bus Selector1/1 -> CUSTOM_POINTS_SIGNALS_RESET_3/2  "<Flag_In_Scope[0|1]>"
  Bus Selector1/13 -> CUSTOM_POINTS_SIGNALS_RESET_3/14  "<Data_3[]>"
  ResetPulse[0|1]/1 -> CUSTOM_POINTS_SIGNALS_RESET_3/1
  Bus Selector1/5 -> CUSTOM_POINTS_SIGNALS_RESET_3/6  "<v_CoorSys_S[m|s]>"
  Bus Selector1/6 -> CUSTOM_POINTS_SIGNALS_RESET_3/7  "<a_CoorSys_S[m|s2]>"
  Bus Selector1/12 -> CUSTOM_POINTS_SIGNALS_RESET_3/13  "<Data_2[]>"
  Bus Selector1/14 -> CUSTOM_POINTS_SIGNALS_RESET_3/15  "<Data_4[]>"
  Bus Selector1/15 -> CUSTOM_POINTS_SIGNALS_RESET_3/16  "<Data_5[]>"
  Bus Selector1/11 -> CUSTOM_POINTS_SIGNALS_RESET_3/12  "<Data_1[]>"
  Bus Selector1/4 -> CUSTOM_POINTS_SIGNALS_RESET_3/5  "<Dist_CoorSys_S[m]>"
  Bus Selector1/10 -> CUSTOM_POINTS_SIGNALS_RESET_3/11  "<Angle_Ver_CoorSys_S[deg]>"
  Bus Selector1/7 -> CUSTOM_POINTS_SIGNALS_RESET_3/8  "<Pos_CoorSys_S[x;y;z][m]>"
  Bus Selector1/8 -> CUSTOM_POINTS_SIGNALS_RESET_3/9  "<Pos_CoorSys_E[x;y;z][m]>"
  Bus Selector1/2 -> CUSTOM_POINTS_SIGNALS_RESET_3/3  "<Flag_Is_Occluded[0|1]>"
  Bus Selector1/9 -> CUSTOM_POINTS_SIGNALS_RESET_3/10  "<Angle_Hor_CoorSys_S[deg]>"
  CustomPoints_Signals_In[]/1 -> Bus Selector1/1

== system ASM_Traffic_V2X_Complete_Model_2/MDL/Environment/Traffic/Sensors/Object_Sensor_3D/CustomPoints/Sensor3/CustomPointsOutput/ResetPulse1 ==
  Enable[0|1] : Inport
  SensorActive[0|1] : Inport  Port=2
  Compare To Constant : simulink/Logic and Bit Operations/Compare To Constant  relop===  const=1  OutDataTypeStr=boolean
  Compare To Constant1 : simulink/Logic and Bit Operations/Compare To Constant  relop===  const=0  OutDataTypeStr=boolean
  Logical Operator1 : Logic  AllPortsSameDT=off  OutDataTypeStr=boolean
  Logical Operator2 : Logic  Operator=NAND  AllPortsSameDT=off  OutDataTypeStr=boolean
  Memory1 : Memory
  ResetPulse[0|1] : Outport
  wires:
  Enable[0|1]/1 -> Logical Operator2/2
  Compare To Constant1/1 -> Logical Operator1/2
  Compare To Constant/1 -> Logical Operator1/1
  Logical Operator1/1 -> ResetPulse[0|1]/1
  SensorActive[0|1]/1 -> Logical Operator2/1
  Logical Operator2/1 -> Memory1/1, Compare To Constant/1
  Memory1/1 -> Compare To Constant1/1

== system ASM_Traffic_V2X_Complete_Model_2/MDL/Environment/Traffic/Sensors/Object_Sensor_3D/CustomPoints/Sensor3/CustomPointsOutput/SignalBus ==
  CustomPoints_Signals_In[] : Inport
  Bus Creator : BusCreator  Inputs=5
  Bus Selector1 : BusSelector  OutputSignals=ID[],Object_ID[],Dist_CoorSys_S[m],Angle_Hor_CoorSys_S[deg],Pos_CoorSys_E[x;y;z][m]
  CustomPoints_Signals_Out[] : Outport
  wires:
  CustomPoints_Signals_In[]/1 -> Bus Selector1/1
  Bus Creator/1 -> CustomPoints_Signals_Out[]/1
  Bus Selector1/4 -> Bus Creator/4  "<Angle_Hor_CoorSys_S[deg]>"
  Bus Selector1/5 -> Bus Creator/5  "<Pos_CoorSys_E[x;y;z][m]>"
  Bus Selector1/2 -> Bus Creator/2  "<Object_ID[]>"
  Bus Selector1/3 -> Bus Creator/3  "<Dist_CoorSys_S[m]>"
  Bus Selector1/1 -> Bus Creator/1  "<ID[]>"

== system ASM_Traffic_V2X_Complete_Model_2/MDL/Environment/Traffic/Sensors/Object_Sensor_3D/RadarEffects/Sensor1/RadarEffectsOutput/HoldSignals ==
  ResetPulse[0|1] : Inport
  RadarEffect_Signals_In[] : Inport  Port=2
  Enable : EnablePort
  Bus Selector1 : BusSelector  OutputSignals=ID[],Dist_CoorSys_S[m],v_CoorSys_S[m|s],Angle_Hor_CoorSys_S[deg],Angle_Ver_CoorSys_S[deg],RCS[dBm2],Object_ID[],Object_Type[],Pos_ObjectPoint_CoorSys_E[x;y;z][m],Pos_ObjectPoint_CoorSys_S[x;y;z][m]
  RADAR_SIGNALS_RESET_1 : ASM_Traffic_lib/Sensors/RadarEffects/RADAR_SIGNALS_RESET  ASMProperties=struct('Name','RADAR_SIGNALS_RESET','Version','1.0','Library','ASM_Traffic_lib')  ASMInstanceName=radar_signals_reset  ASMInstanceID=1
  RadarEffect_Signals_Out[] : Outport
  wires:
  ResetPulse[0|1]/1 -> RADAR_SIGNALS_RESET_1/1
  RADAR_SIGNALS_RESET_1/1 -> RadarEffect_Signals_Out[]/1
  Bus Selector1/3 -> RADAR_SIGNALS_RESET_1/4  "<v_CoorSys_S[m|s]>"
  Bus Selector1/2 -> RADAR_SIGNALS_RESET_1/3  "<Dist_CoorSys_S[m]>"
  Bus Selector1/7 -> RADAR_SIGNALS_RESET_1/8  "<Object_ID[]>"
  Bus Selector1/6 -> RADAR_SIGNALS_RESET_1/7  "<RCS[dBm2]>"
  Bus Selector1/4 -> RADAR_SIGNALS_RESET_1/5  "<Angle_Hor_CoorSys_S[deg]>"
  Bus Selector1/1 -> RADAR_SIGNALS_RESET_1/2  "<ID[]>"
  Bus Selector1/9 -> RADAR_SIGNALS_RESET_1/10  "<Pos_ObjectPoint_CoorSys_E[x;y;z][m]>"
  Bus Selector1/5 -> RADAR_SIGNALS_RESET_1/6  "<Angle_Ver_CoorSys_S[deg]>"
  Bus Selector1/8 -> RADAR_SIGNALS_RESET_1/9  "<Object_Type[]>"
  Bus Selector1/10 -> RADAR_SIGNALS_RESET_1/11  "<Pos_ObjectPoint_CoorSys_S[x;y;z][m]>"
  RadarEffect_Signals_In[]/1 -> Bus Selector1/1
